simulink model "Walk_efficient"  (R2025b)
settings: Solver=VariableStepAuto  StartTime=0.0  StopTime=150  RelTol=0.01  AbsTol=0.01  EnableMultiTasking=on
undefined symbols (not defined in the file): dz, X, Y, Z
libraries: sm_lib x60, nesl_utility x13
(part 3 of 3)

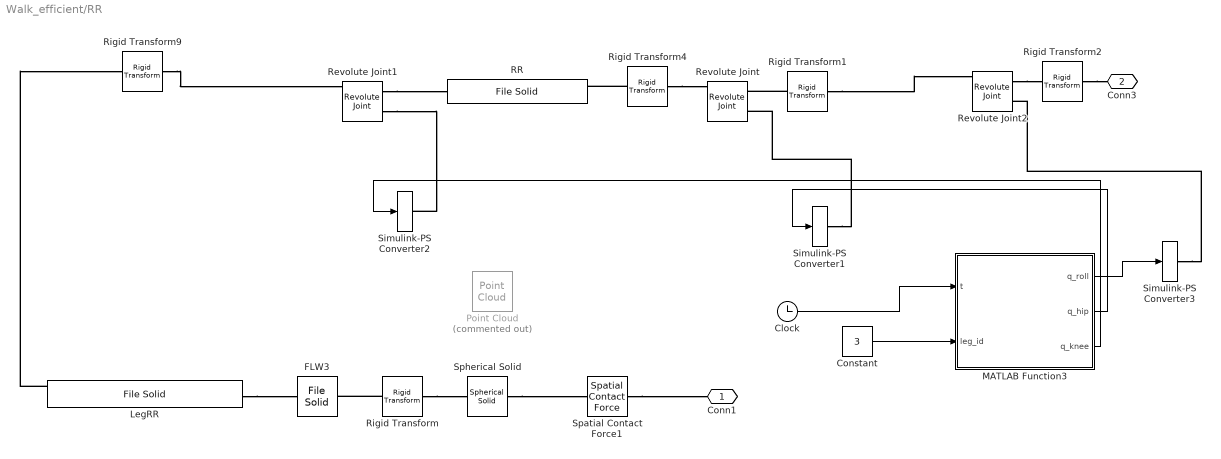
== system Walk_efficient/RR ==
  Clock : Clock
  Constant : Constant  Value=3
  FLW3 : sm_lib/Body Elements/File Solid  ExtGeomFileName=Cheng Shin C-166-1.stp  UnitType=FromFile  ExtGeomFileUnits=m  StepReaderType=HEX  ExportConvexHullGeometry=off  InertiaType=CalculateFromGeometry  BasedOnType=Density  Density=400  DensityUnits=kg/m^3  Mass=1  MassUnits=kg  CenterOfMass=[0 0 0]  CenterOfMassUnits=m  MomentsOfInertia=[1 1 1]  MomentsOfInertiaUnits=kg*m^2  ProductsOfInertia=[0 0 0]  ProductsOfInertiaUnits=kg*m^2  GraphicType=FromGeometry  MarkerShape=Sphere  MarkerSize=10  GraphicVisPropType=AdvancedVisualProperties  GraphicDiffuseColor=[0.1 0.1 0.1]  GraphicOpacity=1  GraphicSpecularColor=[0.2 0.2 0.2 1.0]  GraphicAmbientColor=[0.05 0.05 0.05 1.0]  GraphicEmissiveColor=[0.0 0.0 0.0 1.0]  GraphicShininess=10  DoExposeReferenceFrame=off  SerializedFrames=<Frames><Frame><Id>Frame1</Id><Value><Name>F1</Name><Origin><Source>GeometricFeature</Source><FeatureName>toroidal surface 99</FeatureName></Origin><PrimaryAxis><DefinedDirection>+Z</DefinedDirection><Source>ReferenceFrame</Source><SourceDirection>+Z</SourceDirection><FeatureName></FeatureName></PrimaryAxis><SecondaryAxis><DefinedDirection>+X</DefinedDirection><Source>ReferenceFrame</Source><SourceDirection>+X</SourceDirection><FeatureName></FeatureName></SecondaryAxis></Value></Frame><Frame><Id>Frame2</Id><Value><Name>F2</Name><Origin><Source>CenterOfMassFrame</Source><FeatureName></FeatureName></Origin><PrimaryAxis><DefinedDirection>+Z</DefinedDirection><Source>ReferenceFrame</Source><SourceDirection>+Z</SourceDirection><FeatureName></FeatureName></PrimaryAxis><SecondaryAxis><DefinedDirection>+X</DefinedDirection><Source>ReferenceFrame</Source><SourceDirection>+X</SourceDirection><FeatureName></FeatureName></SecondaryAxis></Value></Frame></Frames>
  LegRR : sm_lib/Body Elements/File Solid  ExtGeomFileName=leg.STEP  UnitType=FromFile  ExtGeomFileUnits=m  StepReaderType=HEX  ExportConvexHullGeometry=on  InertiaType=CalculateFromGeometry  BasedOnType=Density  Density=800  DensityUnits=kg/m^3  Mass=1  MassUnits=kg  CenterOfMass=[0 0 0]  CenterOfMassUnits=m  MomentsOfInertia=[1 1 1]  MomentsOfInertiaUnits=kg*m^2  ProductsOfInertia=[0 0 0]  ProductsOfInertiaUnits=kg*m^2  GraphicType=FromGeometry  MarkerShape=Sphere  MarkerSize=10  GraphicVisPropType=AdvancedVisualProperties  GraphicDiffuseColor=[0 0 0]  GraphicOpacity=1  GraphicSpecularColor=[0.9 0.9 0.9 1.0]  GraphicAmbientColor=[0.1 0.1 0.1 1.0]  GraphicEmissiveColor=[0.0 0.0 0.0 1.0]  GraphicShininess=100  DoExposeReferenceFrame=off  SerializedFrames=|
      | <Frames>
      | 
      |   <Frame>
      |     <Id>Frame1</Id>
      |     <Value>
      |       <Name>L-K link</Name>
      |       <Origin>
      |         <Source>GeometricFeature</Source>
      |         <FeatureName>cylindrical surface 6</FeatureName>
      |       </Origin>
      |       <PrimaryAxis>
      |         <DefinedDirection>+Z</DefinedDirection>
      |         <Source>ReferenceFrame</Source>
      |         <SourceDirection>+Z</SourceDirection>
      |         <FeatureName></FeatureName>
      |       </PrimaryAxis>
      |       <SecondaryAxis>
      |         <DefinedDirection>+X</DefinedDirection>
      |         <Source>ReferenceFrame</Source>
      |         <SourceDirection>-X</SourceDirection>
      |         <FeatureName></FeatureName>
      |       </SecondaryAxis>
      |     </Value>
      |   </Frame>
      | 
      |   <Frame>
      |     <Id>Frame2</Id>
      |     <Value>
      |       <Name>L-W link</Name>
      |       <Origin>
      |         <Source>GeometricFeature</Source>
      |         <FeatureName>cylindrical surface 4</FeatureName>
      |       </Origin>
      |       <PrimaryAxis>
      |         <DefinedDirection>+Z</DefinedDirection>
      |         <Source>ReferenceFrame</Source>
      |         <SourceDirection>+Z</SourceDirection>
      |         <FeatureName></FeatureName>
      |       </PrimaryAxis>
      |       <SecondaryAxis>
      |         <DefinedDirection>+X</DefinedDirection>
      |         <Source>ReferenceFrame</Source>
      |         <SourceDirection>-X</SourceDirection>
      |         <FeatureName></FeatureName>
      |       </SecondaryAxis>
      |     </Value>
      |   </Frame>
      | 
      | </Frames>
  MATLAB Function3 : MATLAB Function  TreatAsAtomicUnit=on
  Point Cloud : sm_lib/Curves and Surfaces/Point Cloud  Commented=on  CoordinatesMatrix=P_hull  CoordinatesMatrixUnits=m  GraphicType=MarkerCloud  GraphicSphereRadius=1e-2  GraphicSphereRadiusUnits=m  GraphicVisPropType=SimpleVisualProperties  GraphicDiffuseColor=[0.5 0.5 0.5]  GraphicOpacity=1  GraphicSpecularColor=[0.5 0.5 0.5 1.0]  GraphicAmbientColor=[0.15 0.15 0.15 1.0]  GraphicEmissiveColor=[0.0 0.0 0.0 1.0]  GraphicShininess=75
  RR : sm_lib/Body Elements/File Solid  ExtGeomFileName=haut patte D.STEP  UnitType=FromFile  ExtGeomFileUnits=m  StepReaderType=HEX  ExportConvexHullGeometry=on  InertiaType=CalculateFromGeometry  BasedOnType=Density  Density=800  DensityUnits=kg/m^3  Mass=1  MassUnits=kg  CenterOfMass=[0 0 0]  CenterOfMassUnits=m  MomentsOfInertia=[1 1 1]  MomentsOfInertiaUnits=kg*m^2  ProductsOfInertia=[0 0 0]  ProductsOfInertiaUnits=kg*m^2  GraphicType=FromGeometry  MarkerShape=Sphere  MarkerSize=10  GraphicVisPropType=AdvancedVisualProperties  GraphicDiffuseColor=[0.9 0.9 0.9]  GraphicOpacity=1  GraphicSpecularColor=[0.9 0.9 0.9 1.0]  GraphicAmbientColor=[0.1 0.1 0.1 1.0]  GraphicEmissiveColor=[0.0 0.0 0.0 1.0]  GraphicShininess=100  DoExposeReferenceFrame=off  SerializedFrames=<Frames><Frame><Id>Frame1</Id><Value><Name>H-L link</Name><Origin><Source>GeometricFeature</Source><FeatureName>spherical surface 2</FeatureName></Origin><PrimaryAxis><DefinedDirection>+Z</DefinedDirection><Source>ReferenceFrame</Source><SourceDirection>+Z</SourceDirection><FeatureName></FeatureName></PrimaryAxis><SecondaryAxis><DefinedDirection>+X</DefinedDirection><Source>ReferenceFrame</Source><SourceDirection>-Y</SourceDirection><FeatureName></FeatureName></SecondaryAxis></Value></Frame><Frame><Id>Frame2</Id><Value><Name>L-K link</Name><Origin><Source>GeometricFeature</Source><FeatureName>cylindrical surface 2</FeatureName></Origin><PrimaryAxis><DefinedDirection>+Z</DefinedDirection><Source>ReferenceFrame</Source><SourceDirection>+Z</SourceDirection><FeatureName></FeatureName></PrimaryAxis><SecondaryAxis><DefinedDirection>+X</DefinedDirection><Source>ReferenceFrame</Source><SourceDirection>-Y</SourceDirection><FeatureName></FeatureName></SecondaryAxis></Value></Frame></Frames>
  Revolute Joint : sm_lib/Joints/Revolute Joint  JointMode=Normal  CompositeWrenchDir=FollowerOnBase  CompositeWrenchFrame=BaseFrame  SenseConstraintForce=off  SenseConstraintTorque=off  SenseTotalForce=off  SenseTotalTorque=off  PositionTargetSpecify=off  PositionTargetPriority=High  PositionTargetValue=0  PositionTargetValueUnits=deg  VelocityTargetSpecify=off  VelocityTargetPriority=High  VelocityTargetValue=0  VelocityTargetValueUnits=deg/s  EquilibriumPosition=0  EquilibriumPositionUnits=deg  SpringStiffness=0  SpringStiffnessUnits=N*m/deg  DampingCoefficient=0  DampingCoefficientUnits=N*m/(deg/s)  LowerLimitSpecify=off  LowerLimitBound=-90  LowerLimitBoundUnits=deg  LowerLimitStiffness=1e4  LowerLimitStiffnessUnits=N*m/deg  LowerLimitDamping=10  LowerLimitDampingUnits=N*m/(deg/s)  LowerLimitTransitionRegionWidth=0.1  LowerLimitTransitionRegionWidthUnits=deg  UpperLimitSpecify=off  UpperLimitBound=90  UpperLimitBoundUnits=deg  UpperLimitStiffness=1e4  UpperLimitStiffnessUnits=N*m/deg  UpperLimitDamping=10  UpperLimitDampingUnits=N*m/(deg/s)  UpperLimitTransitionRegionWidth=0.1  UpperLimitTransitionRegionWidthUnits=deg  TorqueActuationMode=ComputedTorque  MotionActuationMode=InputMotion  SensePosition=on  SenseVelocity=on  SenseAcceleration=off  SenseTorqueForce=off  SenseLowerLimitTorqueForce=off  SenseUpperLimitTorqueForce=off
  Revolute Joint1 : sm_lib/Joints/Revolute Joint  JointMode=Normal  CompositeWrenchDir=FollowerOnBase  CompositeWrenchFrame=BaseFrame  SenseConstraintForce=off  SenseConstraintTorque=off  SenseTotalForce=off  SenseTotalTorque=off  PositionTargetSpecify=off  PositionTargetPriority=High  PositionTargetValue=0  PositionTargetValueUnits=deg  VelocityTargetSpecify=off  VelocityTargetPriority=High  VelocityTargetValue=0  VelocityTargetValueUnits=deg/s  EquilibriumPosition=0  EquilibriumPositionUnits=deg  SpringStiffness=0  SpringStiffnessUnits=N*m/deg  DampingCoefficient=0  DampingCoefficientUnits=N*m/(deg/s)  LowerLimitSpecify=off  LowerLimitBound=-90  LowerLimitBoundUnits=deg  LowerLimitStiffness=1e4  LowerLimitStiffnessUnits=N*m/deg  LowerLimitDamping=10  LowerLimitDampingUnits=N*m/(deg/s)  LowerLimitTransitionRegionWidth=0.1  LowerLimitTransitionRegionWidthUnits=deg  UpperLimitSpecify=off  UpperLimitBound=90  UpperLimitBoundUnits=deg  UpperLimitStiffness=1e4  UpperLimitStiffnessUnits=N*m/deg  UpperLimitDamping=10  UpperLimitDampingUnits=N*m/(deg/s)  UpperLimitTransitionRegionWidth=0.1  UpperLimitTransitionRegionWidthUnits=deg  TorqueActuationMode=ComputedTorque  MotionActuationMode=InputMotion  SensePosition=on  SenseVelocity=on  SenseAcceleration=off  SenseTorqueForce=off  SenseLowerLimitTorqueForce=off  SenseUpperLimitTorqueForce=off
  Revolute Joint2 : sm_lib/Joints/Revolute Joint  JointMode=Normal  CompositeWrenchDir=FollowerOnBase  CompositeWrenchFrame=BaseFrame  SenseConstraintForce=off  SenseConstraintTorque=off  SenseTotalForce=off  SenseTotalTorque=off  PositionTargetSpecify=off  PositionTargetPriority=High  PositionTargetValue=0  PositionTargetValueUnits=deg  VelocityTargetSpecify=off  VelocityTargetPriority=High  VelocityTargetValue=0  VelocityTargetValueUnits=deg/s  EquilibriumPosition=0  EquilibriumPositionUnits=deg  SpringStiffness=0  SpringStiffnessUnits=N*m/deg  DampingCoefficient=0  DampingCoefficientUnits=N*m/(deg/s)  LowerLimitSpecify=off  LowerLimitBound=-90  LowerLimitBoundUnits=deg  LowerLimitStiffness=1e4  LowerLimitStiffnessUnits=N*m/deg  LowerLimitDamping=10  LowerLimitDampingUnits=N*m/(deg/s)  LowerLimitTransitionRegionWidth=0.1  LowerLimitTransitionRegionWidthUnits=deg  UpperLimitSpecify=off  UpperLimitBound=90  UpperLimitBoundUnits=deg  UpperLimitStiffness=1e4  UpperLimitStiffnessUnits=N*m/deg  UpperLimitDamping=10  UpperLimitDampingUnits=N*m/(deg/s)  UpperLimitTransitionRegionWidth=0.1  UpperLimitTransitionRegionWidthUnits=deg  TorqueActuationMode=ComputedTorque  MotionActuationMode=InputMotion  SensePosition=on  SenseVelocity=on  SenseAcceleration=off  SenseTorqueForce=off  SenseLowerLimitTorqueForce=off  SenseUpperLimitTorqueForce=off
  Rigid Transform : sm_lib/Frames and Transforms/Rigid Transform  RotationMethod=None  FollAlignAxisA=+X  BaseAlignAxisA=+Y  FollAlignAxisB=+Y  BaseAlignAxisB=+Z  RotationStandardAxis=+Z  RotationAngle=0  RotationAngleUnits=deg  RotationArbitraryAxis=[0 0 1]  RotationSequenceAxes=FollowerAxes  RotationSequence=XYX  RotationSequenceAngles=[0 0 0]  RotationSequenceAnglesUnits=deg  RotationMatrix=[1 0 0;0 1 0;0 0 1]  Quaternion=[1 0 0 0]  TranslationMethod=Cartesian  TranslationCartesianOffset=[0 dz 0]  TranslationCartesianOffsetUnits=m  TranslationStandardAxis=+Z  TranslationStandardOffset=0  TranslationStandardOffsetUnits=m  TranslationROffset=0  TranslationROffsetUnits=m  TranslationThetaOffset=0  TranslationThetaOffsetUnits=deg  TranslationZOffset=0  TranslationZOffsetUnits=m
  Rigid Transform1 : sm_lib/Frames and Transforms/Rigid Transform  RotationMethod=AlignedAxes  FollAlignAxisA=+Z  BaseAlignAxisA=+Y  FollAlignAxisB=+X  BaseAlignAxisB=+X  RotationStandardAxis=+Z  RotationAngle=0  RotationAngleUnits=deg  RotationArbitraryAxis=[0 0 1]  RotationSequenceAxes=FollowerAxes  RotationSequence=XYX  RotationSequenceAngles=[0 0 0]  RotationSequenceAnglesUnits=deg  RotationMatrix=[1 0 0;0 1 0;0 0 1]  Quaternion=[1 0 0 0]  TranslationMethod=None  TranslationCartesianOffset=[0 0 0]  TranslationCartesianOffsetUnits=m  TranslationStandardAxis=+Z  TranslationStandardOffset=0  TranslationStandardOffsetUnits=m  TranslationROffset=0  TranslationROffsetUnits=m  TranslationThetaOffset=0  TranslationThetaOffsetUnits=deg  TranslationZOffset=0  TranslationZOffsetUnits=m
  Rigid Transform2 : sm_lib/Frames and Transforms/Rigid Transform  RotationMethod=AlignedAxes  FollAlignAxisA=+Y  BaseAlignAxisA=+Y  FollAlignAxisB=+Z  BaseAlignAxisB=+X  RotationStandardAxis=+Z  RotationAngle=0  RotationAngleUnits=deg  RotationArbitraryAxis=[0 0 1]  RotationSequenceAxes=FollowerAxes  RotationSequence=XYX  RotationSequenceAngles=[0 0 0]  RotationSequenceAnglesUnits=deg  RotationMatrix=[1 0 0;0 1 0;0 0 1]  Quaternion=[1 0 0 0]  TranslationMethod=None  TranslationCartesianOffset=[0 0 0]  TranslationCartesianOffsetUnits=m  TranslationStandardAxis=+Z  TranslationStandardOffset=0  TranslationStandardOffsetUnits=m  TranslationROffset=0  TranslationROffsetUnits=m  TranslationThetaOffset=0  TranslationThetaOffsetUnits=deg  TranslationZOffset=0  TranslationZOffsetUnits=m
  Rigid Transform4 : sm_lib/Frames and Transforms/Rigid Transform  RotationMethod=RotationSequence  FollAlignAxisA=+X  BaseAlignAxisA=+Y  FollAlignAxisB=+Y  BaseAlignAxisB=+Z  RotationStandardAxis=+Z  RotationAngle=0  RotationAngleUnits=deg  RotationArbitraryAxis=[0 0 1]  RotationSequenceAxes=FollowerAxes  RotationSequence=XYZ  RotationSequenceAngles=[0 0 -60]  RotationSequenceAnglesUnits=deg  RotationMatrix=[1 0 0;0 1 0;0 0 1]  Quaternion=[1 0 0 0]  TranslationMethod=None  TranslationCartesianOffset=[0 0 0]  TranslationCartesianOffsetUnits=m  TranslationStandardAxis=+Z  TranslationStandardOffset=0  TranslationStandardOffsetUnits=m  TranslationROffset=0  TranslationROffsetUnits=m  TranslationThetaOffset=0  TranslationThetaOffsetUnits=deg  TranslationZOffset=0  TranslationZOffsetUnits=m
  Rigid Transform9 : sm_lib/Frames and Transforms/Rigid Transform  RotationMethod=RotationSequence  FollAlignAxisA=+X  BaseAlignAxisA=+Y  FollAlignAxisB=+Y  BaseAlignAxisB=+Z  RotationStandardAxis=+Z  RotationAngle=0  RotationAngleUnits=deg  RotationArbitraryAxis=[0 0 1]  RotationSequenceAxes=FollowerAxes  RotationSequence=XYZ  RotationSequenceAngles=[0 0 -30]  RotationSequenceAnglesUnits=deg  RotationMatrix=[1 0 0;0 1 0;0 0 1]  Quaternion=[1 0 0 0]  TranslationMethod=None  TranslationCartesianOffset=[0 0 0]  TranslationCartesianOffsetUnits=m  TranslationStandardAxis=+Z  TranslationStandardOffset=0  TranslationStandardOffsetUnits=m  TranslationROffset=0  TranslationROffsetUnits=m  TranslationThetaOffset=0  TranslationThetaOffsetUnits=deg  TranslationZOffset=0  TranslationZOffsetUnits=m
  Simulink-PS Converter1 : nesl_utility/Simulink-PS Converter  PhysicalDomain=network_engine_domain  SubClassName=ps_input  LeftPortType=input  RightPortType=output  PseudoPeriodic=off  Frequencies=[]  NoiseDistribution=none  NoiseParameters=[]  Unit=1  AffineConversion=off  FilteringAndDerivatives=filter  SimscapeFilterOrder=2  InputFilterTimeConstant=0.001  UdotUserProvided=0
  Simulink-PS Converter2 : nesl_utility/Simulink-PS Converter  PhysicalDomain=network_engine_domain  SubClassName=ps_input  LeftPortType=input  RightPortType=output  PseudoPeriodic=off  Frequencies=[]  NoiseDistribution=none  NoiseParameters=[]  Unit=1  AffineConversion=off  FilteringAndDerivatives=filter  SimscapeFilterOrder=2  InputFilterTimeConstant=0.001  UdotUserProvided=0
  Simulink-PS Converter3 : nesl_utility/Simulink-PS Converter  PhysicalDomain=network_engine_domain  SubClassName=ps_input  LeftPortType=input  RightPortType=output  PseudoPeriodic=off  Frequencies=[]  NoiseDistribution=none  NoiseParameters=[]  Unit=1  AffineConversion=off  FilteringAndDerivatives=filter  SimscapeFilterOrder=2  InputFilterTimeConstant=0.001  UdotUserProvided=0
  Spatial Contact Force1 : sm_lib/Forces and Torques/Spatial Contact Force  SenseSeparationDistance=off  NormalForceType=SmoothSpringDamper  NormalStiffness=2e4  NormalStiffnessUnits=N/m  NormalDamping=500  NormalDampingUnits=N/(m/s)  NormalTransitionRegionWidth=2e-3  NormalTransitionRegionWidthUnits=m  FrictionType=SmoothStickSlip  CoefficientOfStaticFriction=0.9  CoefficientOfDynamicFriction=0.7  FrictionalCriticalVelocity=1e-3  FrictionalCriticalVelocityUnits=m/s  SenseContactSignal=off  SensePenetrationDepth=off  SenseNormalVelocity=off  SenseTangentialVelocity=off  SensingForceTorqueDirection=BaseOnFollower  SensingForceTorqueResolutionFrame=ContactFrame  SenseNormalForce=off  SenseNormalForceMagnitude=off  SenseNormalTorque=off  SenseFrictionalForce=off  SenseFrictionalForceMagnitude=off  SenseFrictionalTorque=off  SenseTotalForce=off  SenseTotalTorque=off  SenseContactBaseRotation=off  SenseContactBaseTranslation=off  SenseContactFollowerRotation=off  SenseContactFollowerTranslation=off  ZeroCrossDetectContactStartAndEnd=off
  Spherical Solid : sm_lib/Body Elements/Spherical Solid  SphereRadius=R_sphere  SphereRadiusUnits=m  ExportEntireGeometry=on  InertiaType=CalculateFromGeometry  BasedOnType=Density  Density=1000  DensityUnits=kg/m^3  Mass=1  MassUnits=kg  CenterOfMass=[0 0 0]  CenterOfMassUnits=m  MomentsOfInertia=[1 1 1]  MomentsOfInertiaUnits=kg*m^2  ProductsOfInertia=[0 0 0]  ProductsOfInertiaUnits=kg*m^2  GraphicType=FromGeometry  MarkerShape=Sphere  MarkerSize=10  GraphicVisPropType=SimpleVisualProperties  GraphicDiffuseColor=[0.5 0.5 0.5]  GraphicOpacity=1  GraphicSpecularColor=[0.5 0.5 0.5 1.0]  GraphicAmbientColor=[0.15 0.15 0.15 1.0]  GraphicEmissiveColor=[0.0 0.0 0.0 1.0]  GraphicShininess=75  DoExposeReferenceFrame=on  SerializedFrames=<Frames/>
  Conn1 : PMIOPort  Side=Left
  Conn3 : PMIOPort  Port=2  Side=Right
  wires:
  MATLAB Function3/1(q_roll) -> Simulink-PS Converter3/1
  Constant/1 -> MATLAB Function3/2(leg_id)
  Clock/1 -> MATLAB Function3/1(t)
  MATLAB Function3/2(q_hip) -> Simulink-PS Converter1/1
  MATLAB Function3/3(q_knee) -> Simulink-PS Converter2/1
  connections:
  Rigid Transform1/RConn1 -- Revolute Joint/LConn1
  Rigid Transform4/LConn1 -- Revolute Joint/RConn1
  Rigid Transform1/LConn1 -- Revolute Joint2/RConn1
  Spatial Contact Force1/LConn1 -- Conn1/RConn1
  LegRR/RConn1 -- FLW3/LConn1
  Rigid Transform4/RConn1 -- RR/LConn1
  Revolute Joint1/LConn1 -- RR/RConn1
  Rigid Transform9/LConn1 -- Revolute Joint1/RConn1
  LegRR/LConn1 -- Rigid Transform9/RConn1
  Rigid Transform2/LConn1 -- Conn3/RConn1
  Simulink-PS Converter3/RConn1 -- Revolute Joint2/LConn2
  Simulink-PS Converter1/RConn1 -- Revolute Joint/LConn2
  Revolute Joint1/LConn2 -- Simulink-PS Converter2/RConn1
  Revolute Joint2/LConn1 -- Rigid Transform2/RConn1
  Spherical Solid/LConn1 -- Spatial Contact Force1/RConn1
  Rigid Transform/LConn1 -- FLW3/RConn1
  Rigid Transform/RConn1 -- Spherical Solid/RConn1

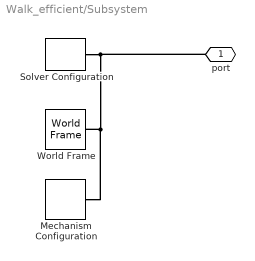
== system Walk_efficient/Subsystem ==
  Mechanism Configuration : sm_lib/Utilities/Mechanism Configuration  UniformGravity=Constant  GravityVector=[0 0 -9.80665]  GravityVectorUnits=m/s^2  LinearizationDelta=0.001  JointModeTransitionNonlinearIterations=2
  Solver Configuration : nesl_utility/Solver Configuration  PhysicalDomain=network_engine_domain  SubClassName=solver  LeftPortType=input  RightPortType=generic  Tones=[]  Harmonics=[]  SimulateNoise=off  Profile=off  UseLocalSampling=off  EnableSwitchedLinearOptims=on  FrequencyDomain=off  UseCCode=off  RelTol=0.001  AbsTol=1e-06  MinStep=1e-09  ToWorkspace=off  RevertToSquareIcSolve=off  NumHomotopyIterations=100  PhasorMode=off  PhasorModeNumHarmonics=1  ConsistencySolver=NEWTON_XTOL_AFTER_FTOL  IndexReductionMethod=DerivativeReplacement  DoDC=off  ResidualTolerance=1e-09  ConsistencyTolSource=GLOBAL  ConsistencyAbsTol=0.001  ConsistencyRelTol=0.001  ConsistencyTolFactor=0.001  UseLocalSolver=off  LocalSolverChoice=NE_BACKWARD_EULER_ADVANCER  ResolveIndetEquations=on  FunctionEvalNumThread=1  LocalSolverSampleTime=0.001  DoFixedCost=off  MaxNonlinIter=3  MaxModeIter=2  ComputeImpulses=off  ImpulseIterations=2  LinearAlgebra=Sparse  LinearAlgebraNumThread=0  EquationFormulation=NE_TIME_EF  DelaysMemoryBudget=1024  AutomaticFiltering=on  FilteringTimeConstant=0.001  PartitionStorageMethod=AS_NEEDED  PartitionMemoryBudget=1024  PartitionMethod=FAST  MultibodyUseLocalSolver=off  MultibodyLocalSolverChoice=ODE1  MultibodyLocalSolverSampleTime=0.001
  World Frame : sm_lib/Frames and Transforms/World Frame
  port : PMIOPort  Side=Right
  connections:
  Solver Configuration/RConn1 -- port/RConn1 -- Mechanism Configuration/RConn1 -- World Frame/RConn1

== matlab function Walk_efficient/RR/MATLAB Function3 ==
  data: t input; q_roll output; leg_id input; q_hip output; q_knee output
function [q_roll, q_hip, q_knee] = motion_walker_v8_extended(t, leg_id)
    % (small stepping + large backward stroke) extended to a complete
    % four-leg cycle
    % Sequence: right front (0) -> left rear (2) -> left front (1) -> right rear (3)
    
    % ================= settings =================
    T_start = 2.0;
    if t < T_start
        q_roll = 0; q_hip = 0; q_knee = 0;
        return;
    end
    t_run = t - T_start;
    
    % [1] Lean(roll) amplitude
    ang_lean = deg2rad(3); 
    
    % [2] Step amplitude (negative value moves forward)
    ang_step = deg2rad(-10); 
    
    % [3] Propulsion amplitude (positive value moves backword)
    ang_push = deg2rad(10);
    
    % [4] Leg lift amplitude
    ang_lift = deg2rad(-12); 
    
    % Period: 4 legs x (2s preparation + 2s action)=16s
    T_cycle = 16.0; 
    tau = mod(t_run, T_cycle);
    
    smooth_move = @(x) (1 - cos(x*pi))/2; 
    lift_arch   = @(x) sin(x*pi);         

    % ================= Logic =================
    q_roll = 0; q_hip = 0; q_knee = 0;
    
    % ---------------------------------------------------------
    % Phase A: Right Front, Leg 0 [0-4s]
    % ---------------------------------------------------------
    if tau < 2.0
        % [Preparation] Shift the center of mass to the left (0 -> -5)
        s = smooth_move(tau/2.0);
        q_roll = s * (-ang_lean);

        
    elseif tau < 4.0
        % [Action] Lift the right front leg
        local_t = (tau - 2.0)/2.0;
        s = smooth_move(local_t);
        q_roll = -ang_lean; % maintain left lean
        
        if leg_id == 0
            % === Main leg: right front leg ===
            q_knee = lift_arch(local_t) * ang_lift;
            q_hip = s * ang_step; 
        else
            % === Supporting legs: other legs ===
            q_knee = 0; 
            q_hip = s * ang_push; % continue backward stroke
        end

    % ---------------------------------------------------------
    % Phase B: Left Rear, Leg 2 [4-8s]
    % ---------------------------------------------------------
    elseif tau < 6.0
        % [Preparation] Shift the center of mass to the right (-5 -> +5)
        local_t = (tau - 4.0)/2.0;
        s = smooth_move(local_t);
        q_roll = -ang_lean + s * (2 * ang_lean);
        
        % Keep the leg that just stepped forward in place; the others keep
        % stroking backward
        if leg_id == 0; q_hip = ang_step; else; q_hip = ang_push; end
        
    elseif tau < 8.0
        % [Action] Lift the left rear leg
        local_t = (tau - 6.0)/2.0;
        s = smooth_move(local_t);
        q_roll = ang_lean; % Maintain right lean
        
        if leg_id == 2
            % === Main leg: left rear leg ===
            q_knee = lift_arch(local_t) * ang_lift;
            q_hip = ang_push + s * (ang_step - ang_push); % Step forward
        else
            % === Supporting legs: other legs ===
            q_knee = 0;
            % Right front leg(0) stays forward, other legs stay backward
            if leg_id == 0; q_hip = ang_step; else; q_hip = ang_push; end
        end

    % ---------------------------------------------------------
    % Phase C: Left Front, Leg 1 [8-12s]
    % ---------------------------------------------------------
    elseif tau < 10.0
         % [Preparation] Keep the center of mass on the right side (no movement)
         % Because the previous motion was the left rear leg (COM on the right),
         % and now the left front leg moves, the COM must remain on the right
        q_roll = ang_lean; 
        
        if leg_id == 0 || leg_id == 2; q_hip = ang_step; else; q_hip = ang_push; end
        
    elseif tau < 12.0
        % [Action] Lift the left front leg
        local_t = (tau - 10.0)/2.0;
        s = smooth_move(local_t);
        q_roll = ang_lean; % Maintain right lean
        
        if leg_id == 1
            % === Main leg: left front leg ===
            q_knee = lift_arch(local_t) * ang_lift;
            q_hip = ang_push + s * (ang_step - ang_push);
        else
            q_knee = 0;
            if leg_id == 0 || leg_id == 2; q_hip = ang_step; else; q_hip = ang_push; end
        end

    % ---------------------------------------------------------
    % Phase D: Right Rear, Leg 3 [12-16s]
    % ---------------------------------------------------------
    elseif tau < 14.0
        % [Preparation] Shift the center of mass from right back to the left (+5 -> -5)
        local_t = (tau - 12.0)/2.0;
        s = smooth_move(local_t);
        q_roll = ang_lean + s * (-2 * ang_lean);
        
        if leg_id == 3; q_hip = ang_push; else; q_hip = ang_step; end
        
    else
        % [Action] Lift the right rear leg
        local_t = (tau - 14.0)/2.0;
        s = smooth_move(local_t);
        q_roll = -ang_lean * (1 - s); % Left lean gradually returns to neutral
        target_pos = 0; 
        if leg_id == 3
            % === Main leg: right rear leg ===
            q_knee = lift_arch(local_t) * ang_lift;
            q_hip = ang_push + s * (target_pos - ang_push);
        else
            q_knee = 0;
            % All other legs return to neutral
            q_hip = ang_step + s * (target_pos - ang_step);
            
        end
    end
end

== matlab function Walk_efficient/FL/MATLAB Function3 ==
  data: t input; q_roll output; leg_id input; q_hip output; q_knee output
function [q_roll, q_hip, q_knee] = motion_walker_v8_extended(t, leg_id)
    % (small stepping + large backward stroke) extended to a complete
    % four-leg cycle
    % Sequence: right front (0) -> left rear (2) -> left front (1) -> right rear (3)
    
    % ================= settings =================
    T_start = 2.0;
    if t < T_start
        q_roll = 0; q_hip = 0; q_knee = 0;
        return;
    end
    t_run = t - T_start;
    
    % [1] Lean(roll) amplitude
    ang_lean = deg2rad(3); 
    
    % [2] Step amplitude (negative value moves forward)
    ang_step = deg2rad(-10); 
    
    % [3] Propulsion amplitude (positive value moves backword)
    ang_push = deg2rad(10);
    
    % [4] Leg lift amplitude
    ang_lift = deg2rad(-12); 
    
    % Period: 4 legs x (2s preparation + 2s action)=16s
    T_cycle = 16.0; 
    tau = mod(t_run, T_cycle);
    
    smooth_move = @(x) (1 - cos(x*pi))/2; 
    lift_arch   = @(x) sin(x*pi);         

    % ================= Logic =================
    q_roll = 0; q_hip = 0; q_knee = 0;
    
    % ---------------------------------------------------------
    % Phase A: Right Front, Leg 0 [0-4s]
    % ---------------------------------------------------------
    if tau < 2.0
        % [Preparation] Shift the center of mass to the left (0 -> -5)
        s = smooth_move(tau/2.0);
        q_roll = s * (-ang_lean);

        
    elseif tau < 4.0
        % [Action] Lift the right front leg
        local_t = (tau - 2.0)/2.0;
        s = smooth_move(local_t);
        q_roll = -ang_lean; % maintain left lean
        
        if leg_id == 0
            % === Main leg: right front leg ===
            q_knee = lift_arch(local_t) * ang_lift;
            q_hip = s * ang_step; 
        else
            % === Supporting legs: other legs ===
            q_knee = 0; 
            q_hip = s * ang_push; % continue backward stroke
        end

    % ---------------------------------------------------------
    % Phase B: Left Rear, Leg 2 [4-8s]
    % ---------------------------------------------------------
    elseif tau < 6.0
        % [Preparation] Shift the center of mass to the right (-5 -> +5)
        local_t = (tau - 4.0)/2.0;
        s = smooth_move(local_t);
        q_roll = -ang_lean + s * (2 * ang_lean);
        
        % Keep the leg that just stepped forward in place; the others keep
        % stroking backward
        if leg_id == 0; q_hip = ang_step; else; q_hip = ang_push; end
        
    elseif tau < 8.0
        % [Action] Lift the left rear leg
        local_t = (tau - 6.0)/2.0;
        s = smooth_move(local_t);
        q_roll = ang_lean; % Maintain right lean
        
        if leg_id == 2
            % === Main leg: left rear leg ===
            q_knee = lift_arch(local_t) * ang_lift;
            q_hip = ang_push + s * (ang_step - ang_push); % Step forward
        else
            % === Supporting legs: other legs ===
            q_knee = 0;
            % Right front leg(0) stays forward, other legs stay backward
            if leg_id == 0; q_hip = ang_step; else; q_hip = ang_push; end
        end

    % ---------------------------------------------------------
    % Phase C: Left Front, Leg 1 [8-12s]
    % ---------------------------------------------------------
    elseif tau < 10.0
         % [Preparation] Keep the center of mass on the right side (no movement)
         % Because the previous motion was the left rear leg (COM on the right),
         % and now the left front leg moves, the COM must remain on the right
        q_roll = ang_lean; 
        
        if leg_id == 0 || leg_id == 2; q_hip = ang_step; else; q_hip = ang_push; end
        
    elseif tau < 12.0
        % [Action] Lift the left front leg
        local_t = (tau - 10.0)/2.0;
        s = smooth_move(local_t);
        q_roll = ang_lean; % Maintain right lean
        
        if leg_id == 1
            % === Main leg: left front leg ===
            q_knee = lift_arch(local_t) * ang_lift;
            q_hip = ang_push + s * (ang_step - ang_push);
        else
            q_knee = 0;
            if leg_id == 0 || leg_id == 2; q_hip = ang_step; else; q_hip = ang_push; end
        end

    % ---------------------------------------------------------
    % Phase D: Right Rear, Leg 3 [12-16s]
    % ---------------------------------------------------------
    elseif tau < 14.0
        % [Preparation] Shift the center of mass from right back to the left (+5 -> -5)
        local_t = (tau - 12.0)/2.0;
        s = smooth_move(local_t);
        q_roll = ang_lean + s * (-2 * ang_lean);
        
        if leg_id == 3; q_hip = ang_push; else; q_hip = ang_step; end
        
    else
        % [Action] Lift the right rear leg
        local_t = (tau - 14.0)/2.0;
        s = smooth_move(local_t);
        q_roll = -ang_lean * (1 - s); % Left lean gradually returns to neutral
        target_pos = 0; 
        if leg_id == 3
            % === Main leg: right rear leg ===
            q_knee = lift_arch(local_t) * ang_lift;
            q_hip = ang_push + s * (target_pos - ang_push);
        else
            q_knee = 0;
            % All other legs return to neutral
            q_hip = ang_step + s * (target_pos - ang_step);
            
        end
    end
end

== matlab function Walk_efficient/FR/MATLAB Function3 ==
  data: t input; q_roll output; leg_id input; q_hip output; q_knee output
function [q_roll, q_hip, q_knee] = motion_walker_v8_extended(t, leg_id)
    % (small stepping + large backward stroke) extended to a complete
    % four-leg cycle
    % Sequence: right front (0) -> left rear (2) -> left front (1) -> right rear (3)
    
    % ================= settings =================
    T_start = 2.0;
    if t < T_start
        q_roll = 0; q_hip = 0; q_knee = 0;
        return;
    end
    t_run = t - T_start;
    
    % [1] Lean(roll) amplitude
    ang_lean = deg2rad(3); 
    
    % [2] Step amplitude (negative value moves forward)
    ang_step = deg2rad(-10); 
    
    % [3] Propulsion amplitude (positive value moves backword)
    ang_push = deg2rad(10);
    
    % [4] Leg lift amplitude
    ang_lift = deg2rad(-12); 
    
    % Period: 4 legs x (2s preparation + 2s action)=16s
    T_cycle = 16.0; 
    tau = mod(t_run, T_cycle);
    
    smooth_move = @(x) (1 - cos(x*pi))/2; 
    lift_arch   = @(x) sin(x*pi);         

    % ================= Logic =================
    q_roll = 0; q_hip = 0; q_knee = 0;
    
    % ---------------------------------------------------------
    % Phase A: Right Front, Leg 0 [0-4s]
    % ---------------------------------------------------------
    if tau < 2.0
        % [Preparation] Shift the center of mass to the left (0 -> -5)
        s = smooth_move(tau/2.0);
        q_roll = s * (-ang_lean);

        
    elseif tau < 4.0
        % [Action] Lift the right front leg
        local_t = (tau - 2.0)/2.0;
        s = smooth_move(local_t);
        q_roll = -ang_lean; % maintain left lean
        
        if leg_id == 0
            % === Main leg: right front leg ===
            q_knee = lift_arch(local_t) * ang_lift;
            q_hip = s * ang_step; 
        else
            % === Supporting legs: other legs ===
            q_knee = 0; 
            q_hip = s * ang_push; % continue backward stroke
        end

    % ---------------------------------------------------------
    % Phase B: Left Rear, Leg 2 [4-8s]
    % ---------------------------------------------------------
    elseif tau < 6.0
        % [Preparation] Shift the center of mass to the right (-5 -> +5)
        local_t = (tau - 4.0)/2.0;
        s = smooth_move(local_t);
        q_roll = -ang_lean + s * (2 * ang_lean);
        
        % Keep the leg that just stepped forward in place; the others keep
        % stroking backward
        if leg_id == 0; q_hip = ang_step; else; q_hip = ang_push; end
        
    elseif tau < 8.0
        % [Action] Lift the left rear leg
        local_t = (tau - 6.0)/2.0;
        s = smooth_move(local_t);
        q_roll = ang_lean; % Maintain right lean
        
        if leg_id == 2
            % === Main leg: left rear leg ===
            q_knee = lift_arch(local_t) * ang_lift;
            q_hip = ang_push + s * (ang_step - ang_push); % Step forward
        else
            % === Supporting legs: other legs ===
            q_knee = 0;
            % Right front leg(0) stays forward, other legs stay backward
            if leg_id == 0; q_hip = ang_step; else; q_hip = ang_push; end
        end

    % ---------------------------------------------------------
    % Phase C: Left Front, Leg 1 [8-12s]
    % ---------------------------------------------------------
    elseif tau < 10.0
         % [Preparation] Keep the center of mass on the right side (no movement)
         % Because the previous motion was the left rear leg (COM on the right),
         % and now the left front leg moves, the COM must remain on the right
        q_roll = ang_lean; 
        
        if leg_id == 0 || leg_id == 2; q_hip = ang_step; else; q_hip = ang_push; end
        
    elseif tau < 12.0
        % [Action] Lift the left front leg
        local_t = (tau - 10.0)/2.0;
        s = smooth_move(local_t);
        q_roll = ang_lean; % Maintain right lean
        
        if leg_id == 1
            % === Main leg: left front leg ===
            q_knee = lift_arch(local_t) * ang_lift;
            q_hip = ang_push + s * (ang_step - ang_push);
        else
            q_knee = 0;
            if leg_id == 0 || leg_id == 2; q_hip = ang_step; else; q_hip = ang_push; end
        end

    % ---------------------------------------------------------
    % Phase D: Right Rear, Leg 3 [12-16s]
    % ---------------------------------------------------------
    elseif tau < 14.0
        % [Preparation] Shift the center of mass from right back to the left (+5 -> -5)
        local_t = (tau - 12.0)/2.0;
        s = smooth_move(local_t);
        q_roll = ang_lean + s * (-2 * ang_lean);
        
        if leg_id == 3; q_hip = ang_push; else; q_hip = ang_step; end
        
    else
        % [Action] Lift the right rear leg
        local_t = (tau - 14.0)/2.0;
        s = smooth_move(local_t);
        q_roll = -ang_lean * (1 - s); % Left lean gradually returns to neutral
        target_pos = 0; 
        if leg_id == 3
            % === Main leg: right rear leg ===
            q_knee = lift_arch(local_t) * ang_lift;
            q_hip = ang_push + s * (target_pos - ang_push);
        else
            q_knee = 0;
            % All other legs return to neutral
            q_hip = ang_step + s * (target_pos - ang_step);
            
        end
    end
end

== matlab function Walk_efficient/RL/MATLAB Function2 ==
  data: t input; q_roll output; leg_id input; q_hip output; q_knee output
function [q_roll, q_hip, q_knee] = motion_walker_v8_extended(t, leg_id)
    % (small stepping + large backward stroke) extended to a complete
    % four-leg cycle
    % Sequence: right front (0) -> left rear (2) -> left front (1) -> right rear (3)
    
    % ================= settings =================
    T_start = 2.0;
    if t < T_start
        q_roll = 0; q_hip = 0; q_knee = 0;
        return;
    end
    t_run = t - T_start;
    
    % [1] Lean(roll) amplitude
    ang_lean = deg2rad(3); 
    
    % [2] Step amplitude (negative value moves forward)
    ang_step = deg2rad(-10); 
    
    % [3] Propulsion amplitude (positive value moves backword)
    ang_push = deg2rad(10);
    
    % [4] Leg lift amplitude
    ang_lift = deg2rad(-12); 
    
    % Period: 4 legs x (2s preparation + 2s action)=16s
    T_cycle = 16.0; 
    tau = mod(t_run, T_cycle);
    
    smooth_move = @(x) (1 - cos(x*pi))/2; 
    lift_arch   = @(x) sin(x*pi);         

    % ================= Logic =================
    q_roll = 0; q_hip = 0; q_knee = 0;
    
    % ---------------------------------------------------------
    % Phase A: Right Front, Leg 0 [0-4s]
    % ---------------------------------------------------------
    if tau < 2.0
        % [Preparation] Shift the center of mass to the left (0 -> -5)
        s = smooth_move(tau/2.0);
        q_roll = s * (-ang_lean);

        
    elseif tau < 4.0
        % [Action] Lift the right front leg
        local_t = (tau - 2.0)/2.0;
        s = smooth_move(local_t);
        q_roll = -ang_lean; % maintain left lean
        
        if leg_id == 0
            % === Main leg: right front leg ===
            q_knee = lift_arch(local_t) * ang_lift;
            q_hip = s * ang_step; 
        else
            % === Supporting legs: other legs ===
            q_knee = 0; 
            q_hip = s * ang_push; % continue backward stroke
        end

    % ---------------------------------------------------------
    % Phase B: Left Rear, Leg 2 [4-8s]
    % ---------------------------------------------------------
    elseif tau < 6.0
        % [Preparation] Shift the center of mass to the right (-5 -> +5)
        local_t = (tau - 4.0)/2.0;
        s = smooth_move(local_t);
        q_roll = -ang_lean + s * (2 * ang_lean);
        
        % Keep the leg that just stepped forward in place; the others keep
        % stroking backward
        if leg_id == 0; q_hip = ang_step; else; q_hip = ang_push; end
        
    elseif tau < 8.0
        % [Action] Lift the left rear leg
        local_t = (tau - 6.0)/2.0;
        s = smooth_move(local_t);
        q_roll = ang_lean; % Maintain right lean
        
        if leg_id == 2
            % === Main leg: left rear leg ===
            q_knee = lift_arch(local_t) * ang_lift;
            q_hip = ang_push + s * (ang_step - ang_push); % Step forward
        else
            % === Supporting legs: other legs ===
            q_knee = 0;
            % Right front leg(0) stays forward, other legs stay backward
            if leg_id == 0; q_hip = ang_step; else; q_hip = ang_push; end
        end

    % ---------------------------------------------------------
    % Phase C: Left Front, Leg 1 [8-12s]
    % ---------------------------------------------------------
    elseif tau < 10.0
         % [Preparation] Keep the center of mass on the right side (no movement)
         % Because the previous motion was the left rear leg (COM on the right),
         % and now the left front leg moves, the COM must remain on the right
        q_roll = ang_lean; 
        
        if leg_id == 0 || leg_id == 2; q_hip = ang_step; else; q_hip = ang_push; end
        
    elseif tau < 12.0
        % [Action] Lift the left front leg
        local_t = (tau - 10.0)/2.0;
        s = smooth_move(local_t);
        q_roll = ang_lean; % Maintain right lean
        
        if leg_id == 1
            % === Main leg: left front leg ===
            q_knee = lift_arch(local_t) * ang_lift;
            q_hip = ang_push + s * (ang_step - ang_push);
        else
            q_knee = 0;
            if leg_id == 0 || leg_id == 2; q_hip = ang_step; else; q_hip = ang_push; end
        end

    % ---------------------------------------------------------
    % Phase D: Right Rear, Leg 3 [12-16s]
    % ---------------------------------------------------------
    elseif tau < 14.0
        % [Preparation] Shift the center of mass from right back to the left (+5 -> -5)
        local_t = (tau - 12.0)/2.0;
        s = smooth_move(local_t);
        q_roll = ang_lean + s * (-2 * ang_lean);
        
        if leg_id == 3; q_hip = ang_push; else; q_hip = ang_step; end
        
    else
        % [Action] Lift the right rear leg
        local_t = (tau - 14.0)/2.0;
        s = smooth_move(local_t);
        q_roll = -ang_lean * (1 - s); % Left lean gradually returns to neutral
        target_pos = 0; 
        if leg_id == 3
            % === Main leg: right rear leg ===
            q_knee = lift_arch(local_t) * ang_lift;
            q_hip = ang_push + s * (target_pos - ang_push);
        else
            q_knee = 0;
            % All other legs return to neutral
            q_hip = ang_step + s * (target_pos - ang_step);
            
        end
    end
end
